simulink library "ftc"  (Simulink 8.1)
settings: Solver=ode45  StartTime=0.0  StopTime=10.0  RelTol=1e-3
undefined symbols (not defined in the file or in its folder): KJUD_BrakeSupportDelay_ms, KJUD_DecelThreshBraking_mps2, KJUD_DriverReactionDelay_ms, KJUD_EarlyTtcDelay_ms, KJUD_FCWActiveDriverDelay_ms, KJUD_FCWAggrDriverDelay_ms, KJUD_FCWConsideredDecel_mps2, KJUD_LateTtcDelay_ms, KJUD_NormalTtcDelay_ms, ZERO_FLOAT
libraries: hcu_lib x1, pbnbs x1, pbbs_new x1
settings Model: Creator=xsellart  LastModifiedBy=tescamilla

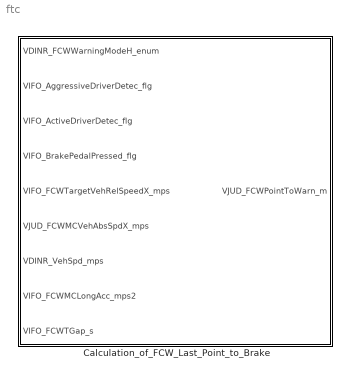
== system ftc ==
  Calculation_of_FCW_Last_Point_to_Brake : Subsystem

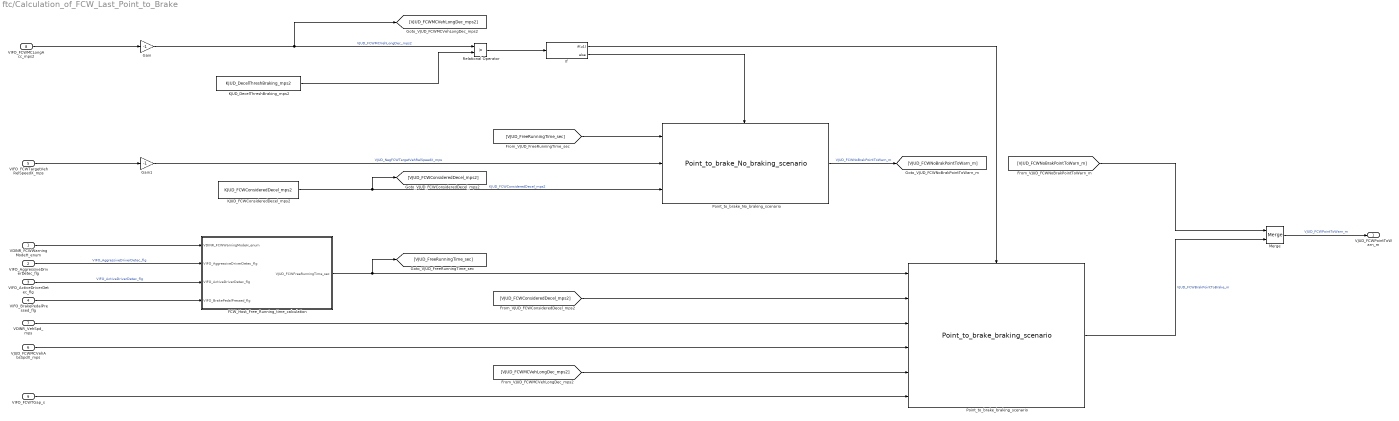
== system ftc/Calculation_of_FCW_Last_Point_to_Brake ==
  VDINR_FCWWarningModeH_enum : Inport
  VIFO_AggressiveDriverDetec_flg : Inport  Port=2
  VIFO_ActiveDriverDetec_flg : Inport  Port=3
  VIFO_BrakePedalPressed_flg : Inport  Port=4
  VIFO_FCWTargetVehRelSpeedX_mps : Inport  Port=5
  VJUD_FCWMCVehAbsSpdX_mps : Inport  Port=6
  VDINR_VehSpd_mps : Inport  Port=7
  VIFO_FCWMCLongAcc_mps2 : Inport  Port=8
  VIFO_FCWTGap_s : Inport  Port=9
  FCW_Host_Free_Running_time_calculation : Subsystem
  Gain : Gain  Gain=-1  OutDataTypeStr=single
  Gain1 : Gain  Gain=-1  OutDataTypeStr=single
  If : If  IfExpression=u1
  KJUD_DecelThreshBraking_mps2 : Constant  Value=KJUD_DecelThreshBraking_mps2  OutDataTypeStr=single
  KJUD_FCWConsideredDecel_mps2 : Constant  Value=KJUD_FCWConsideredDecel_mps2
  Merge : Merge
  Point_to_brake_No_braking_scenario : pbnbs/Point_to_brake_No_braking_scenario
  Point_to_brake_braking_scenario : pbbs_new/Point_to_brake_braking_scenario
  Relational Operator : RelationalOperator  Operator=>  OutDataTypeStr=boolean
  VJUD_FCWPointToWarn_m : Outport
  wires:
  VIFO_AggressiveDriverDetec_flg/1 -> FCW_Host_Free_Running_time_calculation/2(VIFO_AggressiveDriverDetec_flg)  "VIFO_AggressiveDriverDetec_flg"
  VIFO_ActiveDriverDetec_flg/1 -> FCW_Host_Free_Running_time_calculation/3(VIFO_ActiveDriverDetec_flg)  "VIFO_ActiveDriverDetec_flg"
  VIFO_BrakePedalPressed_flg/1 -> FCW_Host_Free_Running_time_calculation/4(VIFO_BrakePedalPressed_flg)
  VIFO_FCWMCLongAcc_mps2/1 -> Gain/1
  KJUD_DecelThreshBraking_mps2/1 -> Relational Operator/2
  VIFO_FCWTargetVehRelSpeedX_mps/1 -> Gain1/1
  Gain/1 -> [VJUD_FCWMCVehLongDec_mps2], Relational Operator/1  "VJUD_FCWMCVehLongDec_mps2"
  Relational Operator/1 -> If/1
  VDINR_VehSpd_mps/1 -> Point_to_brake_braking_scenario/3
  [VJUD_FCWConsideredDecel_mps2] -> Point_to_brake_braking_scenario/2
  VJUD_FCWMCVehAbsSpdX_mps/1 -> Point_to_brake_braking_scenario/4
  FCW_Host_Free_Running_time_calculation/1(VJUD_FCWFreeRunningTime_sec) -> [VJUD_FreeRunningTime_sec], Point_to_brake_braking_scenario/1
  If/1 -> Point_to_brake_braking_scenario/Action
  [VJUD_FCWMCVehLongDec_mps2] -> Point_to_brake_braking_scenario/5
  [VJUD_FreeRunningTime_sec] -> Point_to_brake_No_braking_scenario/1
  Gain1/1 -> Point_to_brake_No_braking_scenario/2  "VJUD_NegFCWTargetVehRelSpeedX_mps"
  KJUD_FCWConsideredDecel_mps2/1 -> [VJUD_FCWConsideredDecel_mps2], Point_to_brake_No_braking_scenario/3  "KJUD_FCWConsideredDecel_mps2"
  If/2 -> Point_to_brake_No_braking_scenario/Action
  Point_to_brake_No_braking_scenario/1 -> [VJUD_FCWNoBrakPointToWarn_m]  "VJUD_FCWNoBrakPointToWarn_m"
  [VJUD_FCWNoBrakPointToWarn_m] -> Merge/1
  Point_to_brake_braking_scenario/1 -> Merge/2  "VJUD_FCWBrakPointToBrake_m"
  Merge/1 -> VJUD_FCWPointToWarn_m/1  "VJUD_FCWPointToWarn_m"
  VDINR_FCWWarningModeH_enum/1 -> FCW_Host_Free_Running_time_calculation/1(VDINR_FCWWarningModeH_enum)
  VIFO_FCWTGap_s/1 -> Point_to_brake_braking_scenario/6

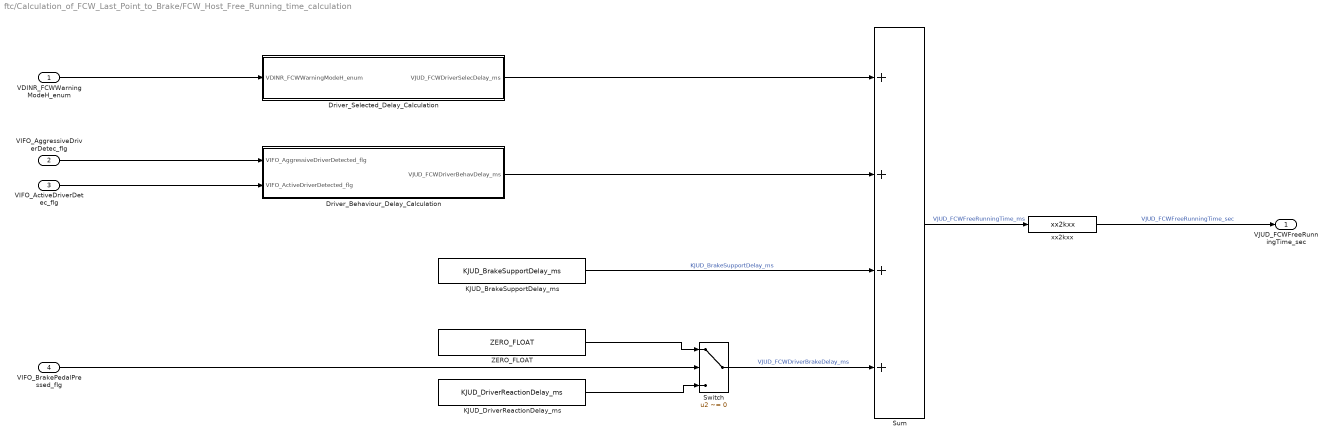
== system ftc/Calculation_of_FCW_Last_Point_to_Brake/FCW_Host_Free_Running_time_calculation ==
  VDINR_FCWWarningModeH_enum : Inport
  VIFO_AggressiveDriverDetec_flg : Inport  Port=2
  VIFO_ActiveDriverDetec_flg : Inport  Port=3
  VIFO_BrakePedalPressed_flg : Inport  Port=4
  Driver_Behaviour_Delay_Calculation : Subsystem
  Driver_Selected_Delay_Calculation : Subsystem
  KJUD_BrakeSupportDelay_ms : Constant  Value=KJUD_BrakeSupportDelay_ms
  KJUD_DriverReactionDelay_ms : Constant  Value=KJUD_DriverReactionDelay_ms
  Sum : Sum  Inputs=++++
  Switch : Switch  Criteria=u2 ~= 0
  ZERO_FLOAT : Constant  Value=ZERO_FLOAT  OutDataTypeStr=single
  xx2kxx : hcu_lib/xx2kxx
  VJUD_FCWFreeRunningTime_sec : Outport
  wires:
  VIFO_AggressiveDriverDetec_flg/1 -> Driver_Behaviour_Delay_Calculation/1(VIFO_AggressiveDriverDetected_flg)
  VDINR_FCWWarningModeH_enum/1 -> Driver_Selected_Delay_Calculation/1(VDINR_FCWWarningModeH_enum)
  VIFO_ActiveDriverDetec_flg/1 -> Driver_Behaviour_Delay_Calculation/2(VIFO_ActiveDriverDetected_flg)
  Driver_Behaviour_Delay_Calculation/1(VJUD_FCWDriverBehavDelay_ms) -> Sum/2
  Driver_Selected_Delay_Calculation/1(VJUD_FCWDriverSelecDelay_ms) -> Sum/1
  KJUD_DriverReactionDelay_ms/1 -> Switch/3
  KJUD_BrakeSupportDelay_ms/1 -> Sum/3  "KJUD_BrakeSupportDelay_ms"
  Sum/1 -> xx2kxx/1  "VJUD_FCWFreeRunningTime_ms"
  ZERO_FLOAT/1 -> Switch/1
  Switch/1 -> Sum/4  "VJUD_FCWDriverBrakeDelay_ms"
  VIFO_BrakePedalPressed_flg/1 -> Switch/2
  xx2kxx/1 -> VJUD_FCWFreeRunningTime_sec/1  "VJUD_FCWFreeRunningTime_sec"

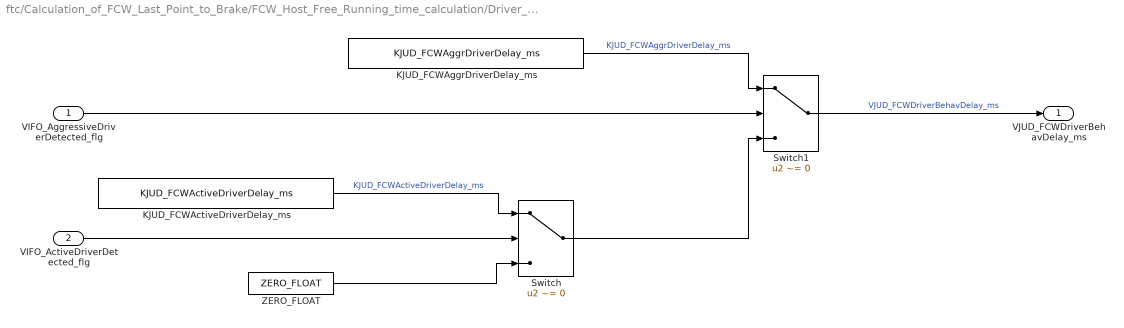
== system ftc/Calculation_of_FCW_Last_Point_to_Brake/FCW_Host_Free_Running_time_calculation/Driver_Behaviour_Delay_Calculation ==
  VIFO_AggressiveDriverDetected_flg : Inport
  VIFO_ActiveDriverDetected_flg : Inport  Port=2
  KJUD_FCWActiveDriverDelay_ms : Constant  Value=KJUD_FCWActiveDriverDelay_ms  OutDataTypeStr=single
  KJUD_FCWAggrDriverDelay_ms : Constant  Value=KJUD_FCWAggrDriverDelay_ms  OutDataTypeStr=single
  Switch : Switch  Criteria=u2 ~= 0
  Switch1 : Switch  Criteria=u2 ~= 0
  ZERO_FLOAT : Constant  Value=ZERO_FLOAT  OutDataTypeStr=single
  VJUD_FCWDriverBehavDelay_ms : Outport
  wires:
  KJUD_FCWAggrDriverDelay_ms/1 -> Switch1/1  "KJUD_FCWAggrDriverDelay_ms"
  Switch/1 -> Switch1/3
  VIFO_AggressiveDriverDetected_flg/1 -> Switch1/2
  KJUD_FCWActiveDriverDelay_ms/1 -> Switch/1  "KJUD_FCWActiveDriverDelay_ms"
  ZERO_FLOAT/1 -> Switch/3
  Switch1/1 -> VJUD_FCWDriverBehavDelay_ms/1  "VJUD_FCWDriverBehavDelay_ms"
  VIFO_ActiveDriverDetected_flg/1 -> Switch/2

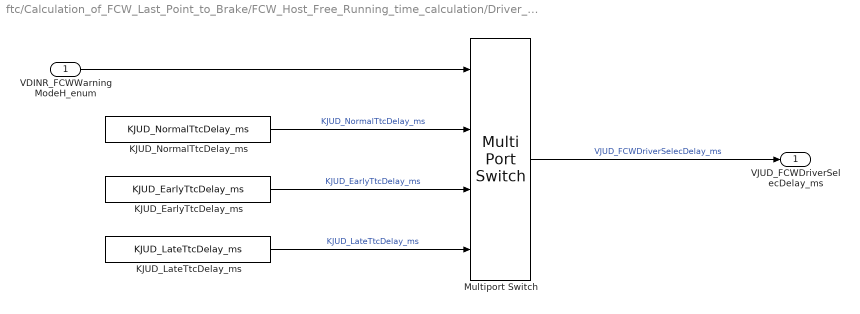
== system ftc/Calculation_of_FCW_Last_Point_to_Brake/FCW_Host_Free_Running_time_calculation/Driver_Selected_Delay_Calculation ==
  VDINR_FCWWarningModeH_enum : Inport
  KJUD_EarlyTtcDelay_ms : Constant  Value=KJUD_EarlyTtcDelay_ms  OutDataTypeStr=single
  KJUD_LateTtcDelay_ms : Constant  Value=KJUD_LateTtcDelay_ms  OutDataTypeStr=single
  KJUD_NormalTtcDelay_ms : Constant  Value=KJUD_NormalTtcDelay_ms  OutDataTypeStr=single
  Multiport Switch : MultiPortSwitch  DataPortOrder=Zero-based contiguous
  VJUD_FCWDriverSelecDelay_ms : Outport
  wires:
  KJUD_LateTtcDelay_ms/1 -> Multiport Switch/4  "KJUD_LateTtcDelay_ms"
  KJUD_EarlyTtcDelay_ms/1 -> Multiport Switch/3  "KJUD_EarlyTtcDelay_ms"
  KJUD_NormalTtcDelay_ms/1 -> Multiport Switch/2  "KJUD_NormalTtcDelay_ms"
  Multiport Switch/1 -> VJUD_FCWDriverSelecDelay_ms/1  "VJUD_FCWDriverSelecDelay_ms"
  VDINR_FCWWarningModeH_enum/1 -> Multiport Switch/1
